simulink library "adc_converter"  (R2023b)
settings: Solver=VariableStepAuto  StartTime=0.0  StopTime=10.0  RelTol=1e-3
undefined symbols (not defined in the file): adc_conv, LowerUserTemp
settings Model: Creator=mueller.chris-it22  LastModifiedBy=mueller.chris-it22

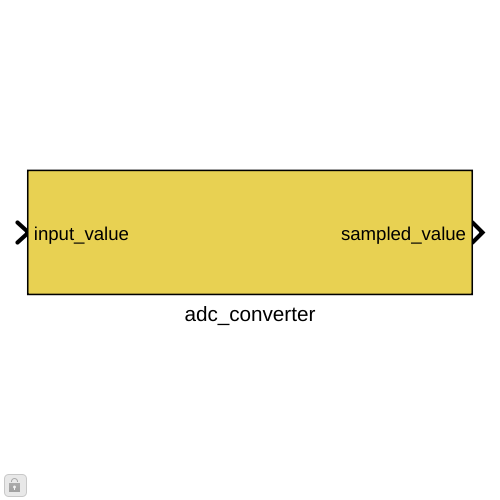
[thumbnail: Simulink's stored preview of the top-level diagram]
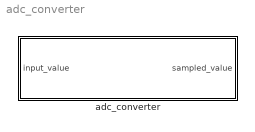
== system adc_converter ==
  adc_converter : Subsystem

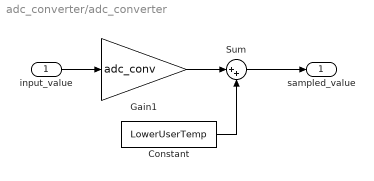
== system adc_converter/adc_converter ==
  input_value : Inport
  Constant : Constant  Value=LowerUserTemp  OutDataTypeStr=uint16
  Gain1 : Gain  Gain=adc_conv  OutDataTypeStr=uint16
  Sum : Sum  Inputs=|++
  sampled_value : Outport
  wires:
  Gain1/1 -> Sum/1
  input_value/1 -> Gain1/1
  Constant/1 -> Sum/2
  Sum/1 -> sampled_value/1
